simulink model "DCMotor"  (Simulink 7.4)
settings: Solver=ode1  StartTime=0.0  StopTime=inf  FixedStep=0.01  RelTol=1e-3
PostLoadFcn:
  | , if any(exist('dsrtsu_mdlpostloadfcn', 'file') == [2, 3, 6]), try dsrtsu_mdlpostloadfcn('Execute', bdroot); catch fprintf('Error in PostLoadFcn (dsrtsu_mdlpostloadfcn) for model "%s":\n %s\n', bdroot, lasterr); end, end,
settings Model: DSRTSU_INTERNAL_RTI_VER=370  DSRTSU_INTERNAL_RTI_TYPE=rti1006  Creator=SE  LastModifiedBy=SE  BufferReuse=off
settings OptimizationCC: BlockReduction=off  OptimizeBlockIOStorage=off  BufferReuse=off  ExpressionFolding=off  LocalBlockOutputs=off  SimCompilerOptimization=On
settings HardwareCC: ProdIntDivRoundTo=Zero  ProdEndianess=LittleEndian  ProdHWDeviceType=Generic->Custom  TargetIntDivRoundTo=Zero  TargetEndianess=LittleEndian  TargetHWDeviceType=Generic->Custom
settings RTWCC: SystemTargetFile=NIVeriStand.tlc  TemplateMakefile=NIVeriStand_vc.tmf  Description=NI VeriStand Real-Time Target for Release 2007b or later  ProcessScript=NIVeriStand_make_rtw_hook
settings STFCustomTargetCC: GeneratePreprocessorConditionals=Disable all  MatFileLogging=on  SystemTargetFile=NIVeriStand.tlc
settings CustomProperty: Value=on
settings EnumStrPairs: String=Default

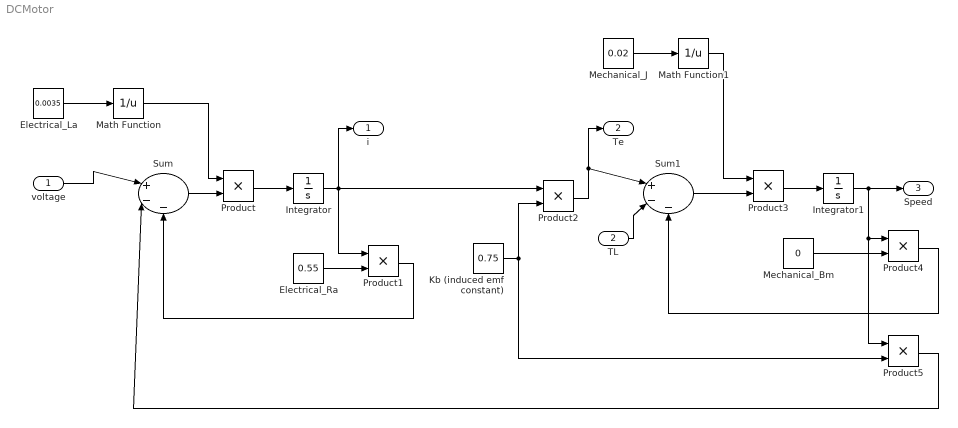
== system DCMotor ==
  voltage : Inport  OutDataType=fixdt(1, 16)  OutScaling=2^0
  TL : Inport  Port=2  OutDataType=fixdt(1, 16)  OutScaling=2^0
  Electrical_La : Constant  Value=0.0035  OutDataType=fixdt(1, 16)  OutScaling=2^0
  Electrical_Ra : Constant  Value=0.55  OutDataType=fixdt(1, 16)  OutScaling=2^0
  Integrator : Integrator
  Integrator1 : Integrator
  Kb (induced emf constant) : Constant  Value=0.75  OutDataType=fixdt(1, 16)  OutScaling=2^0
  Math Function : Math  Operator=reciprocal  OutDataType=fixdt(1, 16)  OutScaling=2^0  SaturateOnIntegerOverflow=on
  Math Function1 : Math  Operator=reciprocal  OutDataType=fixdt(1, 16)  OutScaling=2^0  SaturateOnIntegerOverflow=on
  Mechanical_Bm : Constant  Value=0  OutDataType=fixdt(1, 16)  OutScaling=2^0
  Mechanical_J : Constant  Value=0.02  OutDataType=fixdt(1, 16)  OutScaling=2^0
  Product{,1..5} (6 alike) : Product  OutDataType=fixdt(1, 16)  OutScaling=2^0  RndMeth=Zero
  Sum : Sum  Inputs=|+--  OutDataType=fixdt(1, 16)  OutScaling=2^0
  Sum1 : Sum  Inputs=|+--  OutDataType=fixdt(1, 16)  OutScaling=2^0
  i : Outport  OutDataType=fixdt(1, 16)  OutScaling=2^0
  Te : Outport  Port=2  OutDataType=fixdt(1, 16)  OutScaling=2^0
  Speed : Outport  Port=3  OutDataType=fixdt(1, 16)  OutScaling=2^0
  wires:
  voltage/1 -> Sum/1
  Electrical_La/1 -> Math Function/1
  Math Function/1 -> Product/1
  Sum/1 -> Product/2
  Product/1 -> Integrator/1
  Integrator/1 -> i/1, Product1/1, Product2/1
  Electrical_Ra/1 -> Product1/2
  Product1/1 -> Sum/3
  Kb (induced emf constant)/1 -> Product2/2, Product5/2
  Product2/1 -> Sum1/1, Te/1
  TL/1 -> Sum1/2
  Mechanical_J/1 -> Math Function1/1
  Math Function1/1 -> Product3/1
  Sum1/1 -> Product3/2
  Product3/1 -> Integrator1/1
  Integrator1/1 -> Speed/1, Product4/1, Product5/1
  Mechanical_Bm/1 -> Product4/2
  Product4/1 -> Sum1/3
  Product5/1 -> Sum/2
